simulink model "clase05012021_2"  (R2020b)
settings: Solver=VariableStepAuto  StartTime=0.0  StopTime=1  RelTol=1e-3
libraries: commdigbbndpm3 x1, commutil2 x1
settings Model: Creator=fernando  LastModifiedBy=fernando

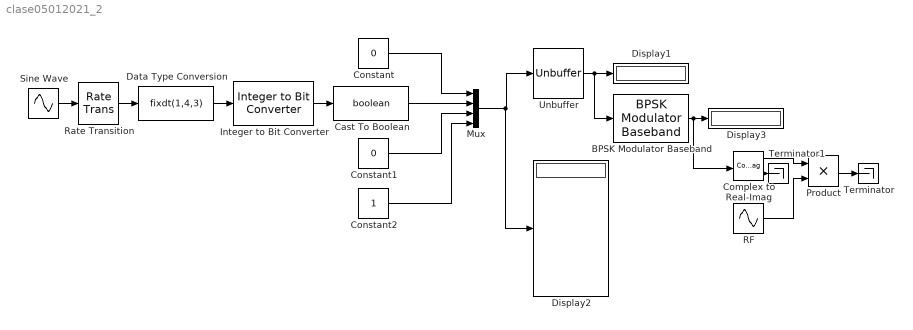
== system clase05012021_2 ==
  BPSK Modulator Baseband : commdigbbndpm3/BPSK Modulator Baseband  Ph=pi  outDtype=double  outWordLen=16  outUDDataType=sfix(16)  outFracLenMode=Best precision  outFracLen=15  outDataTypeStr=double  outLastDataTypeStr=double
      settings: SourceProductName=Communications Toolbox
  Cast To Boolean : DataTypeConversion  OutDataTypeStr=boolean
  Complex to Real-Imag : ComplexToRealImag
  Constant : Constant  Value=0  OutDataTypeStr=boolean
  Constant1 : Constant  Value=0  OutDataTypeStr=boolean
  Constant2 : Constant  OutDataTypeStr=boolean
  Data Type Conversion : DataTypeConversion  OutDataTypeStr=fixdt(1,4,3)
  Display1 : Display
  Display2 : Display
  Display3 : Display
  Integer to Bit Converter : commutil2/Integer to Bit Converter  nbits=4  signedInputValues=Unsigned  bitOrder=MSB first  outDtype=Inherit via internal rule
  Mux : Mux
  Product : Product
  RF : Sin  Frequency=2*pi*140000  SampleTime=0
  Rate Transition : RateTransition  OutPortSampleTime=1/4000
  Sine Wave : Sin  Frequency=2*pi*400  SampleTime=0
  Terminator : Terminator
  Terminator1 : Terminator
  Unbuffer : Unbuffer
  wires:
  Constant2/1 -> Mux/4
  Rate Transition/1 -> Data Type Conversion/1
  Constant1/1 -> Mux/3
  Sine Wave/1 -> Rate Transition/1
  Data Type Conversion/1 -> Integer to Bit Converter/1
  Integer to Bit Converter/1 -> Cast To Boolean/1
  Unbuffer/1 -> BPSK Modulator Baseband/1, Display1/1
  Mux/1 -> Display2/1, Unbuffer/1
  Constant/1 -> Mux/1
  Cast To Boolean/1 -> Mux/2
  BPSK Modulator Baseband/1 -> Complex to Real-Imag/1, Display3/1
  RF/1 -> Product/2
  Product/1 -> Terminator/1
  Complex to Real-Imag/1 -> Product/1
  Complex to Real-Imag/2 -> Terminator1/1
